simulink model "net_model_5_nodes"  (R2024b)
settings: Solver=FixedStepAuto  StartTime=0.0  StopTime=n_max  FixedStep=1  RelTol=1e-3
values from neighbouring files (symbols this model uses):
  A_ctrl = zeros(n, n, n_of_systems)    [compute_controller.m]    (also in compute_controller_sparse.m; controllers.mat = [0.000476978251615 -0.567476341273 -0.00227846807829 0.00303)
  A_matrices = [1 -0.100096864 0 0 0 0.09852592 0 0 0 0.049781138 0.2 0.9633428 ... (900 elements, 10x10x9)]    [ss_matrices_A_conns.mat]
  B = [0 1 0 0 0 0 0 0 0 0 0 0 ... (50 elements, 10x5)]    [ss_matrices_A_conns.mat]
  B_ctrl = -L    [compute_controller.m]    (also in controllers.mat = [0.999523021748 0.0502059606959 0.00227846807829 -0.00303910)
  C = [1 0 0 0 0 0 0 0 0 0 0 1 ... (100 elements, 10x10)]    [ss_matrices_A_conns.mat]
  C_ctrl = J    [compute_controller.m]    (also in controllers.mat = [-0.417173516578 1.38925625612e-17 -0.09852592 -4.1558422613)
  D_ctrl = zeros(m, p, n_of_systems)    [compute_controller.m]    (also in controllers.mat = [0 0 0 0 0 0 0 0 0 0 0 0 ... (450 elements, 5x10x9)])
  K_andrei = balreal(K_final)    [main.m]
  node_1_0 = pi / 180 * [5, 0]'    [main.m]
  node_2_0 = pi / 180 * [-8, 0]'    [main.m]
  node_3_0 = pi / 180 * [2, 0]'    [main.m]
  node_4_0 = pi / 180 * [-8, 0]'    [main.m]
  node_5_0 = pi / 180 * [-3, 0]'    [main.m]
  T_A = zeros(n_states, n_states, n_of_systems)    [compute_controller.m]    (also in controllers.mat = [0.561042741159 -0.215263117802 0.0142825255487 -0.004690356)
  T_B = zeros(n_states, 10, n_of_systems)    [compute_controller.m]    (also in controllers.mat = [-3.4237231262 -3.55838863899 2.62155648543 -1.24980914671 -)
  T_C = zeros(5, n_states, n_of_systems)    [compute_controller.m]    (also in controllers.mat = [-0.00319672869131 -0.042745697524 0.00862967883417 -0.00528)
  T_D = zeros(5, 10, n_of_systems)    [compute_controller.m]    (also in controllers.mat = [0 0 0 0 0 0 0 0 0 0 0 0 ... (450 elements, 5x10x9)])
undefined symbols (not defined in the file or in its folder): a
settings Model: Creator=antoniostavarache  LastModifiedBy=Antonio

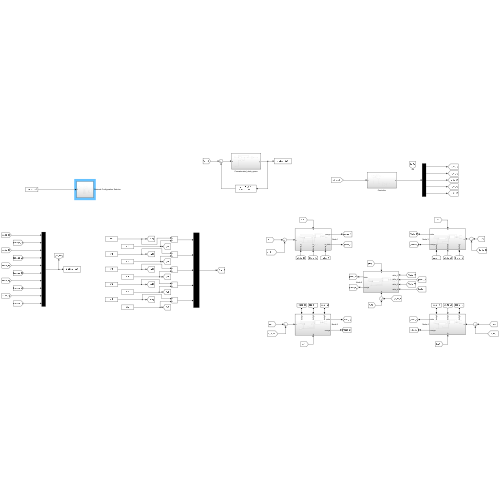
[thumbnail: Simulink's stored preview of the top-level diagram]
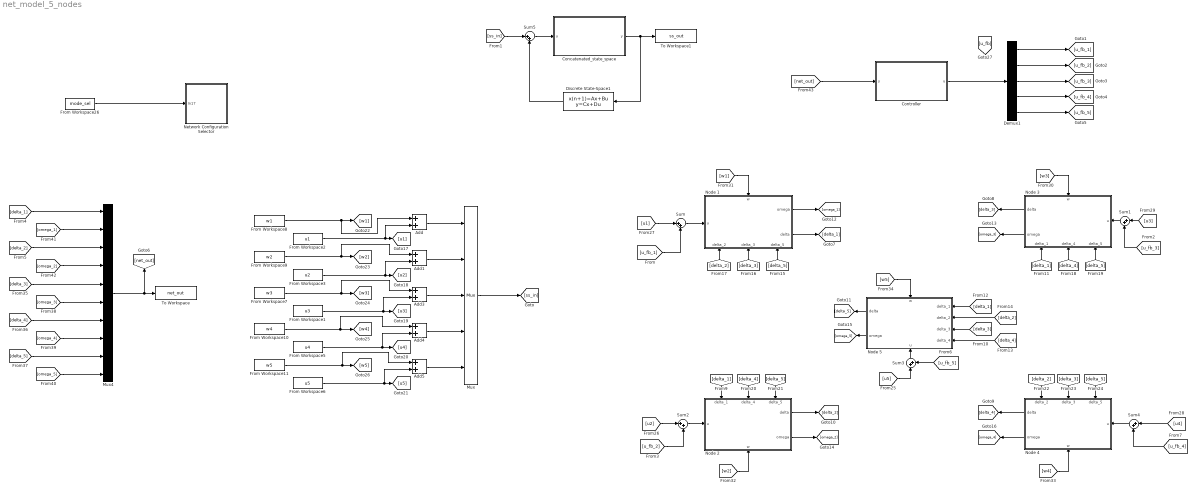
== system net_model_5_nodes ==
  Add{,1,3..5} (5 alike) : Sum
  Concatenated_state_space : Subsystem
  Controller : Subsystem
  Demux1 : Demux  Outputs=5
  Discrete State-Space1 : DiscreteStateSpace  A=K_andrei.A  B=K_andrei.B  C=K_andrei.C  D=K_andrei.D
  From Workspace1 : FromWorkspace  VariableName=u3
  From Workspace10 : FromWorkspace  VariableName=w4
  From Workspace11 : FromWorkspace  VariableName=w5
  From Workspace2 : FromWorkspace  VariableName=u1
  From Workspace26 : FromWorkspace  VariableName=mode_sel
  From Workspace3 : FromWorkspace  VariableName=u2
  From Workspace5 : FromWorkspace  VariableName=u4
  From Workspace6 : FromWorkspace  VariableName=u5
  From Workspace7 : FromWorkspace  VariableName=w3
  From Workspace8 : FromWorkspace  VariableName=w1
  From Workspace9 : FromWorkspace  VariableName=w2
  Mux : Mux  Inputs=5
  Mux4 : Mux  Inputs=10
  Network Configuration Selector : Subsystem
      settings: PortSchema="{\"entries\":[{\"content\":{\"sides\":[{\"content\":{},\"type\":\"ConnectorPlacement.EquallySpacedRectSide\",\"uuid\":\"e46131df-ff90-4f88-82b2-9b0ff679fe5a\"},{\"content\":{\"side\":\"RIGHT\"},\"type\":\"ConnectorPlacement.EquallySpacedRectSide\",\"uuid\":\"3ff9abc5-0c8f-4f25-b3d4-1909347e3840\"},{\"content\":{\"connectorIds\":[\"In1\"],\"side\":\"TOP\"},\"type\":\"ConnectorPlacement.EquallySpacedRectSide\",\"uuid\":\"be576346-0cbc-47fd-9447-c9ae2d46ff4b\"}]},\"type\":\"ConnectorPlacement.EquallySpacedConnector\",\"uuid\":\"fc17ab79-7cb0-4e63-90e3-6a7efbbb7793\"}],\"packageUris\":[\"http://schema.mathworks.com/mf0/Connector/R2020b\"],\"version\":\"1.0\"}"
  Node 1 : Subsystem
      settings: PortSchema="{\"entries\":[{\"content\":{\"sides\":[{\"content\":{\"connectorIds\":[\"In1\"]},\"type\":\"ConnectorPlacement.EquallySpacedRectSide\",\"uuid\":\"cb33889b-91fa-48fc-b9aa-7f1231bd6e44\"},{\"content\":{\"connectorIds\":[\"Out1\",\"Out2\"],\"side\":\"RIGHT\"},\"type\":\"ConnectorPlacement.EquallySpacedRectSide\",\"uuid\":\"1847e095-8e07-44de-8b1e-5e10d245c33d\"},{\"content\":{\"connectorIds\":[\"In2\"],\"side\":\"TOP\"},\"type\":\"ConnectorPlacement.EquallySpacedRectSide\",\"uuid\":\"ffc08770-8d5f-4ddc-b971-47d92d5b44da\"},{\"content\":{\"connectorIds\":[\"In3\",\"In4\",\"In5\"],\"side\":\"BOTTOM\"},\"type\":\"ConnectorPlacement.EquallySpacedRectSide\",\"uuid\":\"a36cd752-5bb5-4dc9-a250-d9ed61d443e3\"}]},\"type\":\"ConnectorPlacement.EquallySpacedConnector\",\"uuid\":\"6b657226-e85b-429c-8361-a0176da114e3\"}],\"packageUris\":[\"http://schema.mathworks.com/mf0/Connector/R2020b\"],\"version\":\"1.0\"}"
  Node 2 : Subsystem
      settings: PortSchema="{\"entries\":[{\"content\":{\"sides\":[{\"content\":{\"connectorIds\":[\"In1\"]},\"type\":\"ConnectorPlacement.EquallySpacedRectSide\",\"uuid\":\"cb33889b-91fa-48fc-b9aa-7f1231bd6e44\"},{\"content\":{\"connectorIds\":[\"Out1\",\"Out2\"],\"side\":\"RIGHT\"},\"type\":\"ConnectorPlacement.EquallySpacedRectSide\",\"uuid\":\"1847e095-8e07-44de-8b1e-5e10d245c33d\"},{\"content\":{\"connectorIds\":[\"In2\",\"In3\",\"In4\"],\"side\":\"TOP\"},\"type\":\"ConnectorPlacement.EquallySpacedRectSide\",\"uuid\":\"ffc08770-8d5f-4ddc-b971-47d92d5b44da\"},{\"content\":{\"connectorIds\":[\"In5\"],\"side\":\"BOTTOM\"},\"type\":\"ConnectorPlacement.EquallySpacedRectSide\",\"uuid\":\"abd9672a-41f4-446f-97bf-4441aa7133ef\"}]},\"type\":\"ConnectorPlacement.EquallySpacedConnector\",\"uuid\":\"6b657226-e85b-429c-8361-a0176da114e3\"}],\"packageUris\":[\"http://schema.mathworks.com/mf0/Connector/R2020b\"],\"version\":\"1.0\"}"
  Node 3 : Subsystem
      settings: PortSchema="{\"entries\":[{\"content\":{\"sides\":[{\"content\":{\"connectorIds\":[\"In1\"]},\"type\":\"ConnectorPlacement.EquallySpacedRectSide\",\"uuid\":\"cb33889b-91fa-48fc-b9aa-7f1231bd6e44\"},{\"content\":{\"connectorIds\":[\"Out1\",\"Out2\"],\"side\":\"RIGHT\"},\"type\":\"ConnectorPlacement.EquallySpacedRectSide\",\"uuid\":\"1847e095-8e07-44de-8b1e-5e10d245c33d\"},{\"content\":{\"connectorIds\":[\"In2\"],\"side\":\"TOP\"},\"type\":\"ConnectorPlacement.EquallySpacedRectSide\",\"uuid\":\"ffc08770-8d5f-4ddc-b971-47d92d5b44da\"},{\"content\":{\"connectorIds\":[\"In3\",\"In4\",\"In5\"],\"side\":\"BOTTOM\"},\"type\":\"ConnectorPlacement.EquallySpacedRectSide\",\"uuid\":\"0b132b39-45cb-4c85-ac05-bcd9e83e299a\"}]},\"type\":\"ConnectorPlacement.EquallySpacedConnector\",\"uuid\":\"6b657226-e85b-429c-8361-a0176da114e3\"}],\"packageUris\":[\"http://schema.mathworks.com/mf0/Connector/R2020b\"],\"version\":\"1.0\"}"
  Node 4 : Subsystem
      settings: PortSchema="{\"entries\":[{\"content\":{\"sides\":[{\"content\":{\"connectorIds\":[\"In1\"]},\"type\":\"ConnectorPlacement.EquallySpacedRectSide\",\"uuid\":\"cb33889b-91fa-48fc-b9aa-7f1231bd6e44\"},{\"content\":{\"connectorIds\":[\"Out1\",\"Out2\"],\"side\":\"RIGHT\"},\"type\":\"ConnectorPlacement.EquallySpacedRectSide\",\"uuid\":\"1847e095-8e07-44de-8b1e-5e10d245c33d\"},{\"content\":{\"connectorIds\":[\"In2\",\"In3\",\"In4\"],\"side\":\"TOP\"},\"type\":\"ConnectorPlacement.EquallySpacedRectSide\",\"uuid\":\"ffc08770-8d5f-4ddc-b971-47d92d5b44da\"},{\"content\":{\"connectorIds\":[\"In5\"],\"side\":\"BOTTOM\"},\"type\":\"ConnectorPlacement.EquallySpacedRectSide\",\"uuid\":\"08756968-8d4f-44c2-a595-fc3b1c48e2ca\"}]},\"type\":\"ConnectorPlacement.EquallySpacedConnector\",\"uuid\":\"6b657226-e85b-429c-8361-a0176da114e3\"}],\"packageUris\":[\"http://schema.mathworks.com/mf0/Connector/R2020b\"],\"version\":\"1.0\"}"
  Node 5 : Subsystem
      settings: PortSchema="{\"entries\":[{\"content\":{\"sides\":[{\"content\":{\"connectorIds\":[\"In1\",\"In2\",\"In3\",\"In4\"]},\"type\":\"ConnectorPlacement.EquallySpacedRectSide\",\"uuid\":\"cb33889b-91fa-48fc-b9aa-7f1231bd6e44\"},{\"content\":{\"connectorIds\":[\"Out1\",\"Out2\"],\"side\":\"RIGHT\"},\"type\":\"ConnectorPlacement.EquallySpacedRectSide\",\"uuid\":\"1847e095-8e07-44de-8b1e-5e10d245c33d\"},{\"content\":{\"connectorIds\":[\"In5\"],\"side\":\"TOP\"},\"type\":\"ConnectorPlacement.EquallySpacedRectSide\",\"uuid\":\"ffc08770-8d5f-4ddc-b971-47d92d5b44da\"},{\"content\":{\"connectorIds\":[\"In6\"],\"side\":\"BOTTOM\"},\"type\":\"ConnectorPlacement.EquallySpacedRectSide\",\"uuid\":\"a3a48786-903f-4ca7-9204-e5bb087ad0f8\"}]},\"type\":\"ConnectorPlacement.EquallySpacedConnector\",\"uuid\":\"6b657226-e85b-429c-8361-a0176da114e3\"}],\"packageUris\":[\"http://schema.mathworks.com/mf0/Connector/R2020b\"],\"version\":\"1.0\"}"
  Sum{,1..5} (6 alike) : Sum  Inputs=|++
  To Workspace : ToWorkspace  VariableName=net_out  SaveFormat=Timeseries  SampleTime=-1
  To Workspace1 : ToWorkspace  VariableName=ss_out  SaveFormat=Timeseries  SampleTime=-1
  wires:
  Node 1/2(delta) -> [delta_1]
  Node 3/1(delta) -> [delta_3]
  [delta_3] -> Node 5/3(delta_3)
  [delta_1] -> Node 3/5(delta_1)
  [delta_1] -> Node 2/2(delta_1)
  [delta_1] -> Node 5/1(delta_1)
  Node 4/1(delta) -> [delta_4]
  [delta_4] -> Node 5/4(delta_4)
  Node 2/1(delta) -> [delta_2]
  [delta_2] -> Node 5/2(delta_2)
  Node 5/1(delta) -> [delta_5]
  [delta_5] -> Node 1/5(delta_5)
  [delta_2] -> Node 1/3(delta_2)
  [delta_3] -> Node 1/4(delta_3)
  [delta_4] -> Node 3/4(delta_4)
  [delta_5] -> Node 3/3(delta_5)
  [delta_5] -> Node 4/2(delta_5)
  [delta_3] -> Node 4/3(delta_3)
  [delta_2] -> Node 4/4(delta_2)
  [delta_4] -> Node 2/3(delta_4)
  [delta_5] -> Node 2/4(delta_5)
  [u2] -> Sum2/1
  [u1] -> Sum/1
  [u3] -> Sum1/1
  [w3] -> Node 3/2(w)
  [w1] -> Node 1/2(w)
  [w2] -> Node 2/5(w)
  [w4] -> Node 4/5(w)
  Node 1/1(omega) -> [omega_1]
  Node 3/2(omega) -> [omega_3]
  Node 2/2(omega) -> [omega_2]
  Node 5/2(omega) -> [omega_5]
  Node 4/2(omega) -> [omega_4]
  [w5] -> Node 5/5(w)
  From Workspace2/1 -> Add/2, [u1]
  From Workspace1/1 -> Add3/2, [u3]
  From Workspace6/1 -> Add5/2, [u5]
  From Workspace5/1 -> Add4/2, [u4]
  From Workspace8/1 -> Add/1, [w1]
  From Workspace7/1 -> Add3/1, [w3]
  From Workspace11/1 -> Add5/1, [w5]
  From Workspace10/1 -> Add4/1, [w4]
  [delta_1] -> Mux4/1
  [omega_1] -> Mux4/2
  [delta_2] -> Mux4/3
  [omega_2] -> Mux4/4
  [delta_3] -> Mux4/5
  [omega_3] -> Mux4/6
  [delta_4] -> Mux4/7
  [omega_4] -> Mux4/8
  [delta_5] -> Mux4/9
  [omega_5] -> Mux4/10
  Mux4/1 -> [net_out], To Workspace/1
  From Workspace3/1 -> Add1/2, [u2]
  From Workspace9/1 -> Add1/1, [w2]
  Add/1 -> Mux/1
  Add1/1 -> Mux/2
  Add3/1 -> Mux/3
  Add4/1 -> Mux/4
  Add5/1 -> Mux/5
  Mux/1 -> [ss_in]
  Concatenated_state_space/1(y) -> Discrete State-Space1/1, To Workspace1/1
  From Workspace26/1 -> Network Configuration Selector/1(In17)
  Demux1/1 -> [u_fb_1]
  Demux1/2 -> [u_fb_2]
  Demux1/3 -> [u_fb_3]
  Demux1/4 -> [u_fb_4]
  Demux1/5 -> [u_fb_5]
  Sum/1 -> Node 1/1(u)
  [u_fb_1] -> Sum/2
  [u_fb_3] -> Sum1/2
  Sum1/1 -> Node 3/1(u)
  [u_fb_2] -> Sum2/2
  Sum2/1 -> Node 2/1(u)
  [u5] -> Sum3/1
  Sum3/1 -> Node 5/6(u)
  [u_fb_5] -> Sum3/2
  [u_fb_4] -> Sum4/2
  Sum4/1 -> Node 4/1(u)
  [u4] -> Sum4/1
  [ss_in] -> Sum5/1
  Sum5/1 -> Concatenated_state_space/1(u)
  [net_out] -> Controller/1(y)
  Controller/1(u) -> Demux1/1
  Discrete State-Space1/1 -> Sum5/2

== system net_model_5_nodes/Concatenated_state_space ==
  u : Inport
  Gain : Gain  Gain=B  Multiplication=Matrix(K*u) (u vector)
  Gain1 : Gain  Gain=C  Multiplication=Matrix(K*u) (u vector)
  Memory : Memory  InitialCondition=[node_1_0; node_2_0; node_3_0; node_4_0; node_5_0]
  Product : Product  Multiplication=Matrix(*)
  Sum : Sum  Inputs=|++
  y : Outport
  wires:
  Product/1 -> Sum/1
  Memory/1 -> Gain1/1, Product/2
  Gain1/1 -> y/1
  u/1 -> Gain/1
  Sum/1 -> Memory/1
  Gain/1 -> Sum/2
  [ss_A] -> Product/1

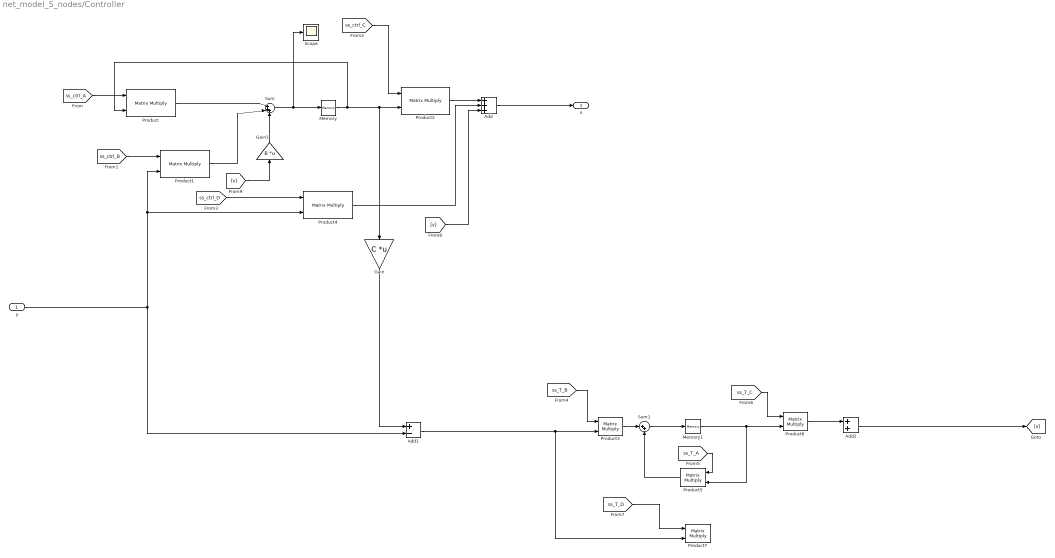
== system net_model_5_nodes/Controller ==
  y : Inport
  Add : Sum  Inputs=+++
  Add1 : Sum  Inputs=+-
  Add2 : Sum
  Gain : Gain  Gain=C  Multiplication=Matrix(K*u) (u vector)
  Gain1 : Gain  Gain=B  Multiplication=Matrix(K*u) (u vector)
  Memory : Memory
  Memory1 : Memory
  Product{,1..7} (8 alike) : Product  Multiplication=Matrix(*)
  Scope : Scope
  Sum : Sum  Inputs=|+++
  Sum1 : Sum  Inputs=|++
  u : Outport
  wires:
  Product/1 -> Sum/1
  Memory/1 -> Gain/1, Product2/2, Product/2
  y/1 -> Product4/2, Product1/2, Add1/2
  Sum/1 -> Scope/1, Memory/1
  Product1/1 -> Sum/2
  [ss_ctrl_C] -> Product2/1
  Product2/1 -> Add/1
  [ss_ctrl_A] -> Product/1
  [ss_ctrl_B] -> Product1/1
  Product4/1 -> Add/2
  [ss_ctrl_D] -> Product4/1
  Gain/1 -> Add1/1
  Sum1/1 -> Memory1/1
  Product3/1 -> Sum1/1
  Add1/1 -> Product7/2, Product3/2
  [ss_T_B] -> Product3/1
  Memory1/1 -> Product6/2, Product5/2
  [ss_T_A] -> Product5/1
  Product5/1 -> Sum1/2
  Product6/1 -> Add2/1
  [ss_T_C] -> Product6/1
  [ss_T_D] -> Product7/1
  [v] -> Gain1/1
  Add2/1 -> [v]
  Add/1 -> u/1
  Gain1/1 -> Sum/3
  [v] -> Add/3

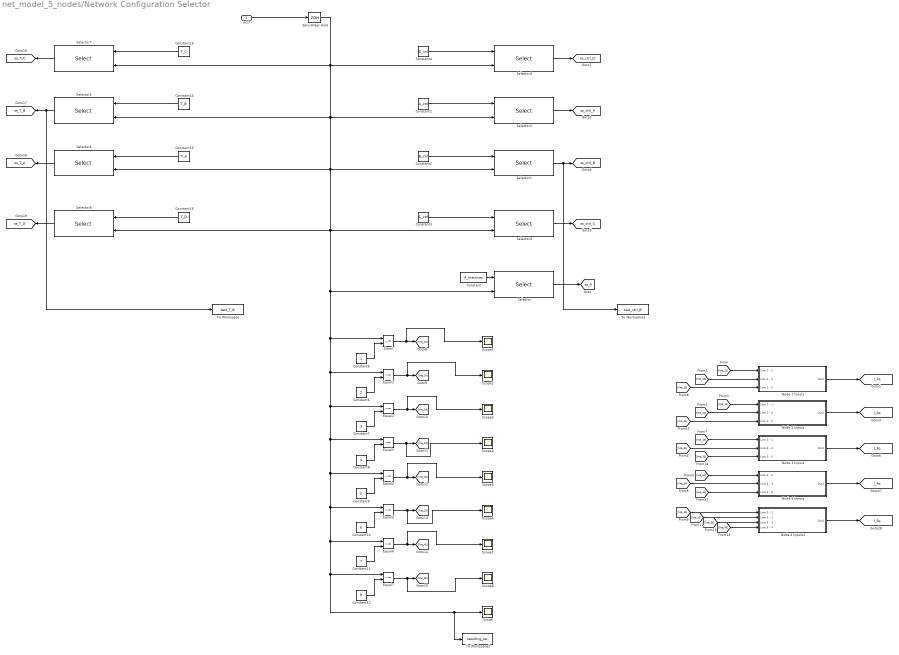
== system net_model_5_nodes/Network Configuration Selector ==
  In17 : Inport
  Constant : Constant  Value=A_matrices
  Constant1 : Constant  Value=A_ctrl  SampleTime=1
  Constant10 : Constant  Value=6
  Constant11 : Constant  Value=7
  Constant12 : Constant  Value=8
  Constant13 : Constant  Value=T_A  SampleTime=1
  Constant14 : Constant  Value=T_B  SampleTime=1
  Constant15 : Constant  Value=T_C  SampleTime=1
  Constant16 : Constant  Value=T_D  SampleTime=1
  Constant2 : Constant  Value=B_ctrl  SampleTime=1
  Constant3 : Constant  Value=C_ctrl  SampleTime=1
  Constant4 : Constant  Value=D_ctrl  SampleTime=1
  Constant5 : Constant
  Constant6 : Constant  Value=2
  Constant7 : Constant  Value=3
  Constant8 : Constant  Value=4
  Constant9 : Constant  Value=5
  Equal{,1..7} (8 alike) : RelationalOperator  Operator=~=  OutDataTypeStr=boolean  RndMeth=Simplest  InputSameDT=off
  Node 1 Inputs : Subsystem
  Node 2 Inputs : Subsystem
  Node 3 Inputs : Subsystem
  Node 4 Inputs : Subsystem
  Node 4 Inputs1 : Subsystem
  Scope{,1..8} (9 alike) : Scope
  Selector{,1..8} (9 alike) : Selector  NumberOfDimensions=3  InputPortWidth=3  IndexOptions=Select all,Select all,Index vector (port)  Indices=a,1,1  OutputSizes=1,1,1
  To Workspace : ToWorkspace  VariableName=test_T_B  SaveFormat=Timeseries  SampleTime=-1
  To Workspace1 : ToWorkspace  VariableName=test_ctrl_B  SaveFormat=Timeseries  SampleTime=-1
  To Workspace2 : ToWorkspace  VariableName=resulting_sw  SaveFormat=Timeseries  SampleTime=-1
  Zero-Order Hold : ZeroOrderHold  SampleTime=5
  tag scope: l_1q=global, l_2q=global, l_3q=global, l_4q=global, l_5q=global, ss_A=global, ss_T_A=global, ss_T_B=global, ss_T_C=global, ss_T_D=global, ss_ctrl_A=global, ss_ctrl_B=global, ss_ctrl_C=global, ss_ctrl_D=global
  wires:
  Node 2 Inputs/1(Out1) -> [l_2q]
  Node 3 Inputs/1(Out1) -> [l_3q]
  Node 4 Inputs1/1(Out1) -> [l_5q]
  Node 1 Inputs/1(Out1) -> [l_1q]
  Node 4 Inputs/1(Out1) -> [l_4q]
  Constant/1 -> Selector/1
  Selector/1 -> [ss_A]
  Selector2/1 -> [ss_ctrl_A]
  Selector1/1 -> To Workspace1/1, [ss_ctrl_B]
  Selector3/1 -> [ss_ctrl_C]
  Constant1/1 -> Selector2/1
  Constant2/1 -> Selector1/1
  Constant3/1 -> Selector3/1
  Constant4/1 -> Selector4/1
  Selector4/1 -> [ss_ctrl_D]
  In17/1 -> Zero-Order Hold/1
  Constant5/1 -> Equal/2
  Equal/1 -> Scope1/1, [line_12]
  [line_12] -> Node 1 Inputs/1(Line 1 - 2)
  [line_12] -> Node 2 Inputs/1(Line 2 - 1)
  Constant6/1 -> Equal1/2
  Equal1/1 -> Scope2/1, [line_24]
  [line_24] -> Node 2 Inputs/2(Line 2 - 4)
  [line_24] -> Node 4 Inputs/1(Line 4 - 2)
  Constant7/1 -> Equal2/2
  [line_34] -> Node 3 Inputs/2(Line 3 - 4)
  [line_34] -> Node 4 Inputs/2(Line 4 - 3)
  Constant8/1 -> Equal3/2
  [line_13] -> Node 1 Inputs/2(Line 1 - 3)
  [line_13] -> Node 3 Inputs/1(Line 3 - 1)
  Constant9/1 -> Equal4/2
  [line_15] -> Node 1 Inputs/3(Line 1 - 5)
  [line_15] -> Node 4 Inputs1/1(Line 5 - 1)
  Constant10/1 -> Equal5/2
  [line_25] -> Node 2 Inputs/3(Line 2 - 5)
  [line_25] -> Node 4 Inputs1/2(Line 5 - 2)
  Constant11/1 -> Equal6/2
  [line_45] -> Node 4 Inputs/3(Line 4 - 5)
  [line_45] -> Node 4 Inputs1/4(Line 5 - 4)
  Constant12/1 -> Equal7/2
  [line_35] -> Node 3 Inputs/3(Line 3 - 5)
  [line_35] -> Node 4 Inputs1/3(Line 5 - 3)
  Equal3/1 -> Scope4/1, [line_13]
  Equal2/1 -> Scope3/1, [line_34]
  Equal5/1 -> Scope6/1, [line_25]
  Equal4/1 -> Scope5/1, [line_15]
  Equal7/1 -> Scope8/1, [line_35]
  Equal6/1 -> Scope7/1, [line_45]
  Zero-Order Hold/1 -> Equal/1, Equal7/1, To Workspace2/1, Scope/1, Equal6/1, Equal5/1, Equal4/1, Equal3/1, Equal2/1, Equal1/1, Selector/2, Selector8/2, Selector3/2, Selector6/2, Selector1/2, Selector5/2, Selector2/2, Selector7/2, Selector4/2
  Constant13/1 -> Selector6/1
  Constant16/1 -> Selector8/1
  Selector8/1 -> [ss_T_D]
  Selector7/1 -> [ss_T_C]
  Constant14/1 -> Selector5/1
  Selector6/1 -> [ss_T_A]
  Constant15/1 -> Selector7/1
  Selector5/1 -> To Workspace/1, [ss_T_B]

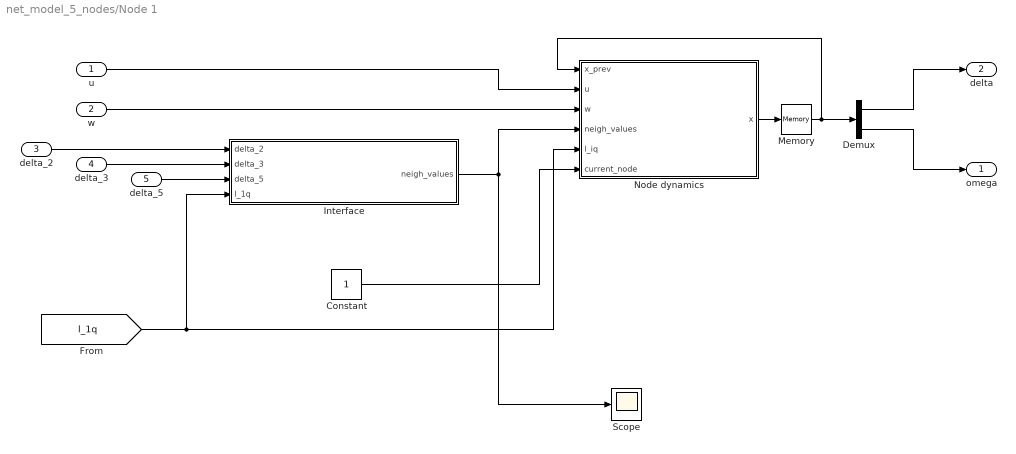
== system net_model_5_nodes/Node 1 ==
  u : Inport
  w : Inport  Port=2
  delta_2 : Inport  Port=3
  delta_3 : Inport  Port=4
  delta_5 : Inport  Port=5
  Constant : Constant
  Demux : Demux  Outputs=2
  Interface : MATLAB Function  TreatAsAtomicUnit=on
  Memory : Memory  InitialCondition=node_1_0
  Node dynamics : MATLAB Function  TreatAsAtomicUnit=on
  Scope : Scope
  omega : Outport
  delta : Outport  Port=2
  wires:
  Node dynamics/1(x) -> Memory/1
  Interface/1(neigh_values) -> Node dynamics/4(neigh_values), Scope/1
  u/1 -> Node dynamics/2(u)
  w/1 -> Node dynamics/3(w)
  Demux/1 -> delta/1
  Demux/2 -> omega/1
  Memory/1 -> Node dynamics/1(x_prev), Demux/1
  delta_2/1 -> Interface/1(delta_2)
  [l_1q] -> Node dynamics/5(l_iq), Interface/4(l_1q)
  Constant/1 -> Node dynamics/6(current_node)
  delta_3/1 -> Interface/2(delta_3)
  delta_5/1 -> Interface/3(delta_5)

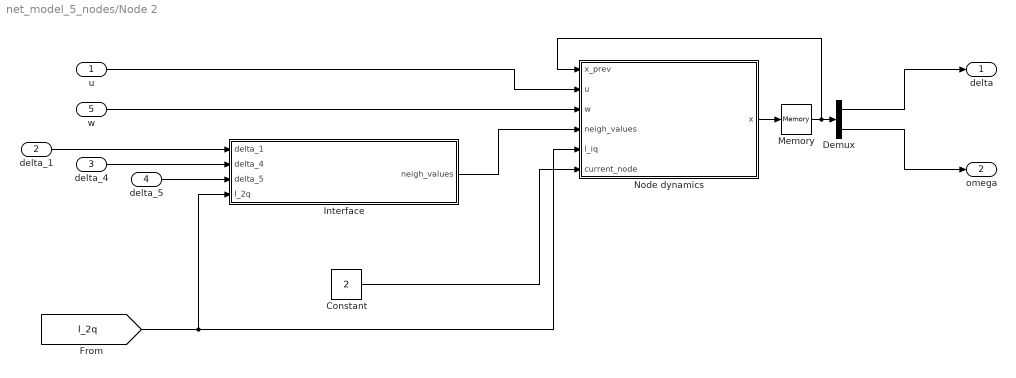
== system net_model_5_nodes/Node 2 ==
  u : Inport
  delta_1 : Inport  Port=2
  delta_4 : Inport  Port=3
  delta_5 : Inport  Port=4
  w : Inport  Port=5
  Constant : Constant  Value=2
  Demux : Demux  Outputs=2
  Interface : MATLAB Function  TreatAsAtomicUnit=on
  Memory : Memory  InitialCondition=node_2_0
  Node dynamics : MATLAB Function  TreatAsAtomicUnit=on
  delta : Outport
  omega : Outport  Port=2
  wires:
  Node dynamics/1(x) -> Memory/1
  Interface/1(neigh_values) -> Node dynamics/4(neigh_values)
  u/1 -> Node dynamics/2(u)
  w/1 -> Node dynamics/3(w)
  Demux/1 -> delta/1
  Demux/2 -> omega/1
  Memory/1 -> Node dynamics/1(x_prev), Demux/1
  delta_1/1 -> Interface/1(delta_1)
  Constant/1 -> Node dynamics/6(current_node)
  [l_2q] -> Interface/4(l_2q), Node dynamics/5(l_iq)
  delta_4/1 -> Interface/2(delta_4)
  delta_5/1 -> Interface/3(delta_5)

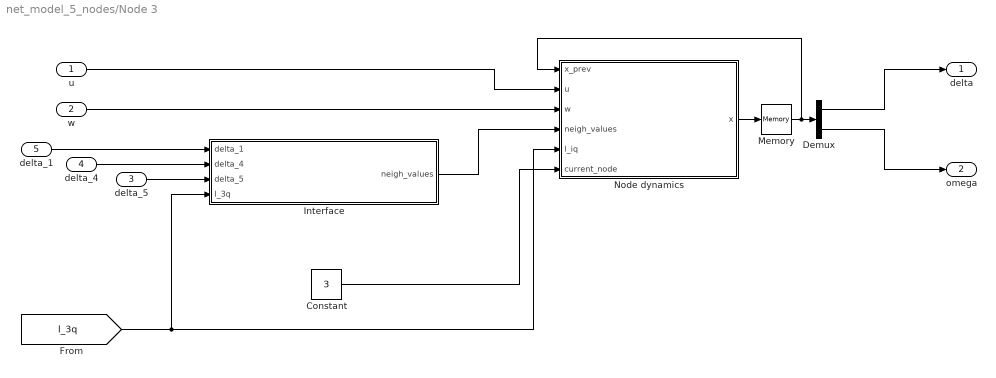
== system net_model_5_nodes/Node 3 ==
  u : Inport
  w : Inport  Port=2
  delta_5 : Inport  Port=3
  delta_4 : Inport  Port=4
  delta_1 : Inport  Port=5
  Constant : Constant  Value=3
  Demux : Demux  Outputs=2
  Interface : MATLAB Function  TreatAsAtomicUnit=on
  Memory : Memory  InitialCondition=node_3_0
  Node dynamics : MATLAB Function  TreatAsAtomicUnit=on
  delta : Outport
  omega : Outport  Port=2
  wires:
  Node dynamics/1(x) -> Memory/1
  Interface/1(neigh_values) -> Node dynamics/4(neigh_values)
  u/1 -> Node dynamics/2(u)
  w/1 -> Node dynamics/3(w)
  Demux/1 -> delta/1
  Demux/2 -> omega/1
  Memory/1 -> Node dynamics/1(x_prev), Demux/1
  delta_1/1 -> Interface/1(delta_1)
  [l_3q] -> Interface/4(l_3q), Node dynamics/5(l_iq)
  Constant/1 -> Node dynamics/6(current_node)
  delta_4/1 -> Interface/2(delta_4)
  delta_5/1 -> Interface/3(delta_5)

== system net_model_5_nodes/Node 4 ==
  u : Inport
  delta_5 : Inport  Port=2
  delta_3 : Inport  Port=3
  delta_2 : Inport  Port=4
  w : Inport  Port=5
  Constant : Constant  Value=4
  Demux : Demux  Outputs=2
  Interface : MATLAB Function  TreatAsAtomicUnit=on
  Memory : Memory  InitialCondition=node_4_0
  Node dynamics : MATLAB Function  TreatAsAtomicUnit=on
  delta : Outport
  omega : Outport  Port=2
  wires:
  Node dynamics/1(x) -> Memory/1
  Interface/1(neigh_values) -> Node dynamics/4(neigh_values)
  u/1 -> Node dynamics/2(u)
  w/1 -> Node dynamics/3(w)
  Demux/1 -> delta/1
  Demux/2 -> omega/1
  Memory/1 -> Node dynamics/1(x_prev), Demux/1
  delta_2/1 -> Interface/1(delta_2)
  [l_4q] -> Interface/4(l_4q), Node dynamics/5(l_iq)
  Constant/1 -> Node dynamics/6(current_node)
  delta_3/1 -> Interface/2(delta_3)
  delta_5/1 -> Interface/3(delta_5)

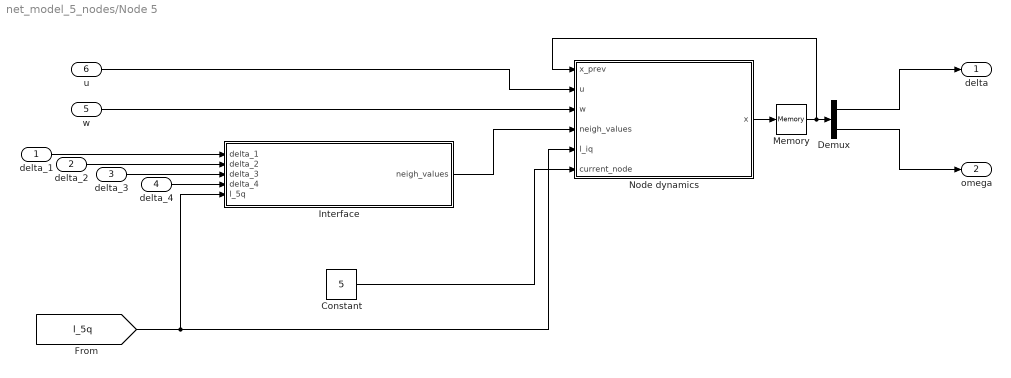
== system net_model_5_nodes/Node 5 ==
  delta_1 : Inport
  delta_2 : Inport  Port=2
  delta_3 : Inport  Port=3
  delta_4 : Inport  Port=4
  w : Inport  Port=5
  u : Inport  Port=6
  Constant : Constant  Value=5
  Demux : Demux  Outputs=2
  Interface : MATLAB Function  TreatAsAtomicUnit=on
  Memory : Memory  InitialCondition=node_5_0
  Node dynamics : MATLAB Function  TreatAsAtomicUnit=on
  delta : Outport
  omega : Outport  Port=2
  wires:
  Node dynamics/1(x) -> Memory/1
  Interface/1(neigh_values) -> Node dynamics/4(neigh_values)
  u/1 -> Node dynamics/2(u)
  w/1 -> Node dynamics/3(w)
  Demux/1 -> delta/1
  Demux/2 -> omega/1
  Memory/1 -> Node dynamics/1(x_prev), Demux/1
  delta_1/1 -> Interface/1(delta_1)
  [l_5q] -> Interface/5(l_5q), Node dynamics/5(l_iq)
  Constant/1 -> Node dynamics/6(current_node)
  delta_2/1 -> Interface/2(delta_2)
  delta_3/1 -> Interface/3(delta_3)
  delta_4/1 -> Interface/4(delta_4)

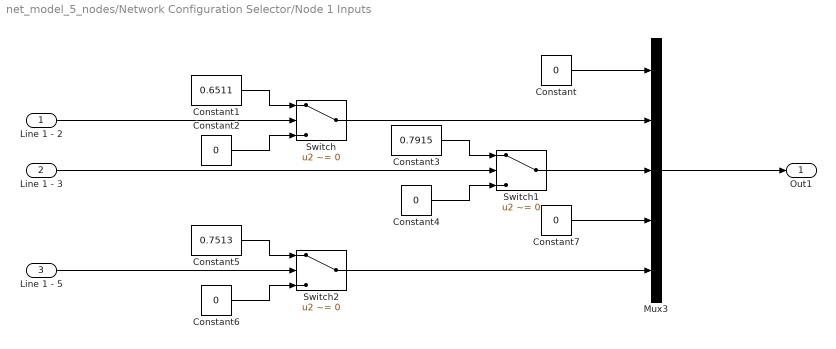
== system net_model_5_nodes/Network Configuration Selector/Node 1 Inputs ==
  Line 1 - 2 : Inport
  Line 1 - 3 : Inport  Port=2
  Line 1 - 5 : Inport  Port=3
  Constant{,2,4,6..7} (5 alike) : Constant  Value=0
  Constant1 : Constant  Value=0.6511
  Constant3 : Constant  Value=0.7915
  Constant5 : Constant  Value=0.7513
  Mux3 : Mux  Inputs=5
  Switch : Switch  Criteria=u2 ~= 0  SaturateOnIntegerOverflow=off  InputSameDT=off
  Switch1 : Switch  Criteria=u2 ~= 0  SaturateOnIntegerOverflow=off  InputSameDT=off
  Switch2 : Switch  Criteria=u2 ~= 0  SaturateOnIntegerOverflow=off  InputSameDT=off
  Out1 : Outport
  wires:
  Mux3/1 -> Out1/1
  Line 1 - 2/1 -> Switch/2
  Constant/1 -> Mux3/1
  Switch/1 -> Mux3/2
  Constant2/1 -> Switch/3
  Constant1/1 -> Switch/1
  Constant3/1 -> Switch1/1
  Line 1 - 3/1 -> Switch1/2
  Constant4/1 -> Switch1/3
  Switch1/1 -> Mux3/3
  Constant6/1 -> Switch2/3
  Line 1 - 5/1 -> Switch2/2
  Constant5/1 -> Switch2/1
  Switch2/1 -> Mux3/5
  Constant7/1 -> Mux3/4

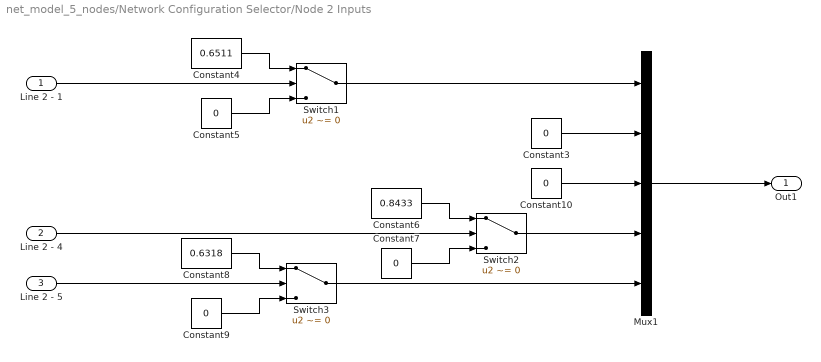
== system net_model_5_nodes/Network Configuration Selector/Node 2 Inputs ==
  Line 2 - 1 : Inport
  Line 2 - 4 : Inport  Port=2
  Line 2 - 5 : Inport  Port=3
  Constant{3,5,7,9..10} (5 alike) : Constant  Value=0
  Constant4 : Constant  Value=0.6511
  Constant6 : Constant  Value=0.8433
  Constant8 : Constant  Value=0.6318
  Mux1 : Mux  Inputs=5
  Switch1 : Switch  Criteria=u2 ~= 0  SaturateOnIntegerOverflow=off  InputSameDT=off
  Switch2 : Switch  Criteria=u2 ~= 0  SaturateOnIntegerOverflow=off  InputSameDT=off
  Switch3 : Switch  Criteria=u2 ~= 0  SaturateOnIntegerOverflow=off  InputSameDT=off
  Out1 : Outport
  wires:
  Constant8/1 -> Switch3/1
  Constant9/1 -> Switch3/3
  Line 2 - 4/1 -> Switch2/2
  Constant7/1 -> Switch2/3
  Constant6/1 -> Switch2/1
  Switch3/1 -> Mux1/5
  Constant4/1 -> Switch1/1
  Line 2 - 1/1 -> Switch1/2
  Constant5/1 -> Switch1/3
  Line 2 - 5/1 -> Switch3/2
  Mux1/1 -> Out1/1
  Switch1/1 -> Mux1/1
  Constant3/1 -> Mux1/2
  Constant10/1 -> Mux1/3
  Switch2/1 -> Mux1/4

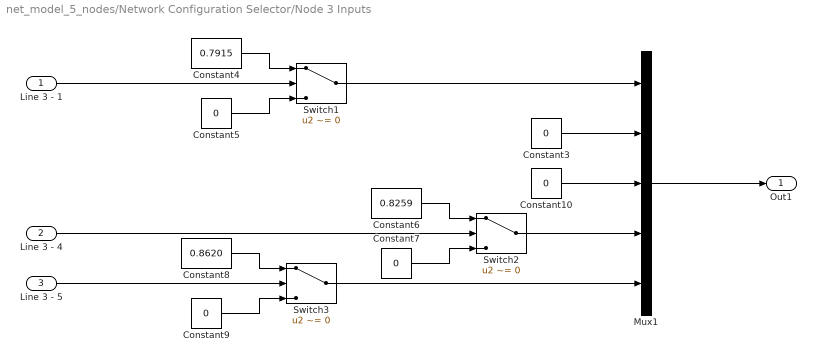
== system net_model_5_nodes/Network Configuration Selector/Node 3 Inputs ==
  Line 3 - 1 : Inport
  Line 3 - 4 : Inport  Port=2
  Line 3 - 5 : Inport  Port=3
  Constant{3,5,7,9..10} (5 alike) : Constant  Value=0
  Constant4 : Constant  Value=0.7915
  Constant6 : Constant  Value=0.8259
  Constant8 : Constant  Value=0.8620
  Mux1 : Mux  Inputs=5
  Switch1 : Switch  Criteria=u2 ~= 0  SaturateOnIntegerOverflow=off  InputSameDT=off
  Switch2 : Switch  Criteria=u2 ~= 0  SaturateOnIntegerOverflow=off  InputSameDT=off
  Switch3 : Switch  Criteria=u2 ~= 0  SaturateOnIntegerOverflow=off  InputSameDT=off
  Out1 : Outport
  wires:
  Line 3 - 1/1 -> Switch1/2
  Line 3 - 5/1 -> Switch3/2
  Constant5/1 -> Switch1/3
  Line 3 - 4/1 -> Switch2/2
  Constant7/1 -> Switch2/3
  Constant4/1 -> Switch1/1
  Constant9/1 -> Switch3/3
  Constant6/1 -> Switch2/1
  Constant10/1 -> Mux1/3
  Mux1/1 -> Out1/1
  Constant8/1 -> Switch3/1
  Switch2/1 -> Mux1/4
  Switch3/1 -> Mux1/5
  Switch1/1 -> Mux1/1
  Constant3/1 -> Mux1/2

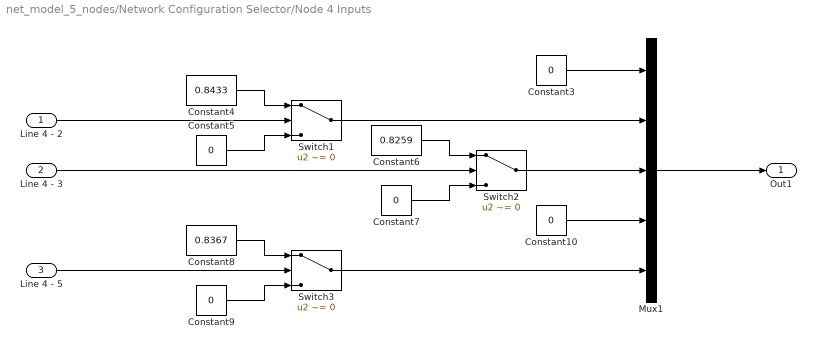
== system net_model_5_nodes/Network Configuration Selector/Node 4 Inputs ==
  Line 4 - 2 : Inport
  Line 4 - 3 : Inport  Port=2
  Line 4 - 5 : Inport  Port=3
  Constant{3,5,7,9..10} (5 alike) : Constant  Value=0
  Constant4 : Constant  Value=0.8433
  Constant6 : Constant  Value=0.8259
  Constant8 : Constant  Value=0.8367
  Mux1 : Mux  Inputs=5
  Switch1 : Switch  Criteria=u2 ~= 0  SaturateOnIntegerOverflow=off  InputSameDT=off
  Switch2 : Switch  Criteria=u2 ~= 0  SaturateOnIntegerOverflow=off  InputSameDT=off
  Switch3 : Switch  Criteria=u2 ~= 0  SaturateOnIntegerOverflow=off  InputSameDT=off
  Out1 : Outport
  wires:
  Mux1/1 -> Out1/1
  Line 4 - 2/1 -> Switch1/2
  Line 4 - 5/1 -> Switch3/2
  Constant5/1 -> Switch1/3
  Switch3/1 -> Mux1/5
  Constant8/1 -> Switch3/1
  Constant9/1 -> Switch3/3
  Constant7/1 -> Switch2/3
  Constant4/1 -> Switch1/1
  Constant6/1 -> Switch2/1
  Line 4 - 3/1 -> Switch2/2
  Constant3/1 -> Mux1/1
  Constant10/1 -> Mux1/4
  Switch2/1 -> Mux1/3
  Switch1/1 -> Mux1/2

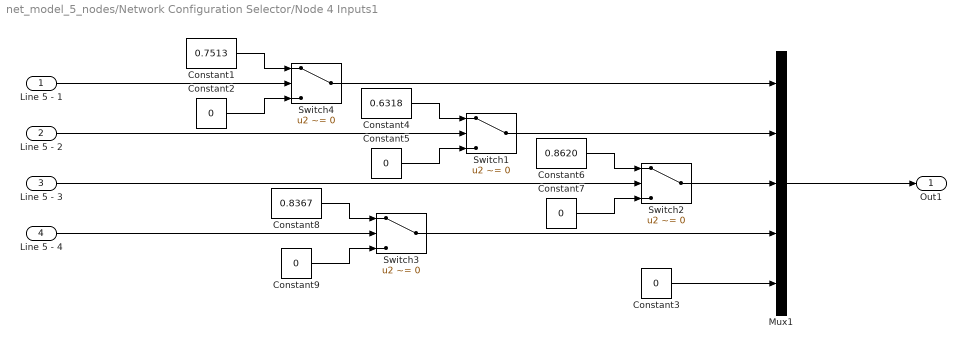
== system net_model_5_nodes/Network Configuration Selector/Node 4 Inputs1 ==
  Line 5 - 1 : Inport
  Line 5 - 2 : Inport  Port=2
  Line 5 - 3 : Inport  Port=3
  Line 5 - 4 : Inport  Port=4
  Constant1 : Constant  Value=0.7513
  Constant{2..3,5,7,9} (5 alike) : Constant  Value=0
  Constant4 : Constant  Value=0.6318
  Constant6 : Constant  Value=0.8620
  Constant8 : Constant  Value=0.8367
  Mux1 : Mux  Inputs=5
  Switch{1..4} (4 alike) : Switch  Criteria=u2 ~= 0  SaturateOnIntegerOverflow=off  InputSameDT=off
  Out1 : Outport
  wires:
  Line 5 - 2/1 -> Switch1/2
  Switch1/1 -> Mux1/2
  Constant7/1 -> Switch2/3
  Constant6/1 -> Switch2/1
  Constant4/1 -> Switch1/1
  Constant9/1 -> Switch3/3
  Constant8/1 -> Switch3/1
  Line 5 - 3/1 -> Switch2/2
  Line 5 - 4/1 -> Switch3/2
  Mux1/1 -> Out1/1
  Constant5/1 -> Switch1/3
  Switch2/1 -> Mux1/3
  Constant1/1 -> Switch4/1
  Constant2/1 -> Switch4/3
  Switch4/1 -> Mux1/1
  Line 5 - 1/1 -> Switch4/2
  Switch3/1 -> Mux1/4
  Constant3/1 -> Mux1/5

== matlab function net_model_5_nodes/Node 5/Interface ==
  data: delta_1 input; neigh_values output; delta_2 input; delta_3 input; delta_4 input; l_5q input
function neigh_values = fcn(delta_1, delta_2, delta_3, delta_4, l_5q)

    neigh_values = l_5q(1) * delta_1 + l_5q(2) * delta_2 + l_5q(3) * delta_3 + l_5q(4) * delta_4;

end

== matlab function net_model_5_nodes/Node 5/Node dynamics ==
  data: x_prev input; u input; x output; w input; neigh_values input; l_iq input; current_node input
function x = fcn(x_prev, u, w, neigh_values, l_iq, current_node)
    
    % current_node = 1;

%%

    hi = [0.3244
        1.5886;
        0.6224;
        1.0571;
        0.3313];

    di = [0.5650;
        0.7844;
        0.7347;
        0.5060;
        0.6686];

    dt = 0.2;
%%

    a21 = -hi(current_node) * dt * sum(l_iq);
    a22 = 1 - hi(current_node) * di(current_node) * dt;

    A = [1, dt;
        a21, a22];

    x = A * x_prev + [0 1]' * (u + w + hi(current_node) * dt * neigh_values);
    
end

== matlab function net_model_5_nodes/Node 1/Interface ==
  data: delta_2 input; delta_3 input; delta_5 input; neigh_values output; l_1q input
function neigh_values = fcn(delta_2, delta_3, delta_5, l_1q)

    neigh_values = l_1q(2) * delta_2 + l_1q(3) * delta_3 + l_1q(5) * delta_5;

end

== matlab function net_model_5_nodes/Node 1/Node dynamics ==
  data: x_prev input; u input; x output; w input; neigh_values input; l_iq input; current_node input
function x = fcn(x_prev, u, w, neigh_values, l_iq, current_node)
    
    % current_node = 1;

%%

    hi = [0.3244
        1.5886;
        0.6224;
        1.0571;
        0.3313];

    di = [0.5650;
        0.7844;
        0.7347;
        0.5060;
        0.6686];

    dt = 0.2;
%%

    a21 = -hi(current_node) * dt * sum(l_iq);
    a22 = 1 - hi(current_node) * di(current_node) * dt;

    A = [1, dt;
        a21, a22];

    x = A * x_prev + [0 1]' * (u + w + hi(current_node) * dt * neigh_values);
    
end

== matlab function net_model_5_nodes/Node 3/Interface ==
  data: delta_1 input; neigh_values output; delta_4 input; delta_5 input; l_3q input
function neigh_values = fcn(delta_1, delta_4, delta_5, l_3q)

    neigh_values = l_3q(1) * delta_1 + l_3q(4) * delta_4 + l_3q(5) * delta_5;

end

== matlab function net_model_5_nodes/Node 3/Node dynamics ==
  data: x_prev input; u input; x output; w input; neigh_values input; l_iq input; current_node input
function x = fcn(x_prev, u, w, neigh_values, l_iq, current_node)
    
    % current_node = 1;

%%

    hi = [0.3244
        1.5886;
        0.6224;
        1.0571;
        0.3313];

    di = [0.5650;
        0.7844;
        0.7347;
        0.5060;
        0.6686];
    dt = 0.2;
%%

    a21 = -hi(current_node) * dt * sum(l_iq);
    a22 = 1 - hi(current_node) * di(current_node) * dt;

    A = [1, dt;
        a21, a22];

    x = A * x_prev + [0 1]' * (u + w + hi(current_node) * dt * neigh_values);
    
end

== matlab function net_model_5_nodes/Node 2/Interface ==
  data: delta_1 input; neigh_values output; delta_4 input; delta_5 input; l_2q input
function neigh_values = fcn(delta_1, delta_4, delta_5, l_2q)

    neigh_values = l_2q(1) * delta_1 + l_2q(4) * delta_4 + l_2q(5) * delta_5;

end

== matlab function net_model_5_nodes/Node 2/Node dynamics ==
  data: x_prev input; u input; x output; w input; neigh_values input; l_iq input; current_node input
function x = fcn(x_prev, u, w, neigh_values, l_iq, current_node)
    
    % current_node = 1;

%%

    hi = [0.3244
        1.5886;
        0.6224;
        1.0571;
        0.3313];

    di = [0.5650;
        0.7844;
        0.7347;
        0.5060;
        0.6686];

    dt = 0.2;
%%

    a21 = -hi(current_node) * dt * sum(l_iq);
    a22 = 1 - hi(current_node) * di(current_node) * dt;

    A = [1, dt;
        a21, a22];

    x = A * x_prev + [0 1]' * (u + w + hi(current_node) * dt * neigh_values);
    
end

== matlab function net_model_5_nodes/Node 4/Interface ==
  data: delta_2 input; neigh_values output; delta_3 input; delta_5 input; l_4q input
function neigh_values = fcn(delta_2, delta_3, delta_5, l_4q)

    neigh_values = l_4q(2) * delta_2 + l_4q(3) * delta_3 + l_4q(5) * delta_5;

end

== matlab function net_model_5_nodes/Node 4/Node dynamics ==
  data: x_prev input; u input; x output; w input; neigh_values input; l_iq input; current_node input
function x = fcn(x_prev, u, w, neigh_values, l_iq, current_node)
    
    % current_node = 1;

%%

    hi = [0.3244
        1.5886;
        0.6224;
        1.0571;
        0.3313];

    di = [0.5650;
        0.7844;
        0.7347;
        0.5060;
        0.6686];

    dt = 0.2;
%%

    a21 = -hi(current_node) * dt * sum(l_iq);
    a22 = 1 - hi(current_node) * di(current_node) * dt;

    A = [1, dt;
        a21, a22];

    x = A * x_prev + [0 1]' * (u + w + hi(current_node) * dt * neigh_values);
    
end
